simulink model "Kubon_lab6_sim_test"  (R2020a)
settings: Solver=VariableStepAuto  StartTime=0.0  StopTime=10  RelTol=1e-3
values from neighbouring files (symbols this model uses):
  a1 = 1    [Kubon_lab4.m]    (also in Kubon_lab6.m = Aw1*sqrt(2*g/H1); Kubon_lab6_test.m = Aw1*sqrt(2*g/H1); Kubon_lab7.m = Aw1*sqrt(2*g/(H1-H2)); Kubon_lab8.m = Aw1*sqrt(2*g/(H1-H2)))
  A1 = [0,-6/7,-16/7,47/7]    [Kubon_lab4.m]    (also in Kubon_lab6.m = 1; Kubon_lab6_test.m = 1; Kubon_lab7.m = 4; Kubon_lab8.m = 4)
  A2 = 7    [Kubon_lab6.m]    (also in Kubon_lab6_test.m; Kubon_lab7.m = 4; Kubon_lab8.m = 4)
  a2 = Aw2*sqrt(2*g/H2)    [Kubon_lab6.m]    (also in Kubon_lab6_test.m; Kubon_lab7.m; Kubon_lab8.m)
  dfwe1 = 0.1*fwe1max    [Kubon_lab6_test.m]
  dfwe2 = 0.1*fwe2max    [Kubon_lab6_test.m]
  fwe1 = fwe1w(i)    [Kubon_lab6.m]    (also in Kubon_lab6_test.m; Kubon_lab7.m = 0.1*fwe1max; Kubon_lab8.m = 0.1*fwe1max)
  fwe2 = fwe2w(i)    [Kubon_lab6.m]    (also in Kubon_lab6_test.m; Kubon_lab7.m; Kubon_lab8.m)
  h10 = fwe1/a1    [Kubon_lab6.m]    (also in Kubon_lab6_test.m; Kubon_lab7.m = (1/(2*g))*(fwe1/Aw1)^2 + (1/(2*g))*(((fwe2+fwe1)/Aw2)^2); Kubon_lab8.m = fwe1/a1+(fwe2+fwe1)/a2)
  h20 = (fwe1+fwe2)/a2    [Kubon_lab6.m]    (also in Kubon_lab6_test.m; Kubon_lab7.m = 1/(2*g)*(((fwe1+fwe2)/Aw2)^2); Kubon_lab8.m = (fwe2+fwe1)/a2)
  t0 = 50.0    (= 50)    [Kubon_lab10.m]    (also in Kubon_lab4.m = 5; Kubon_lab5.m = 0; Kubon_lab6.m = 5; Kubon_lab6_test.m = 0)
settings Model: Creator=dominika  LastModifiedBy=dominika

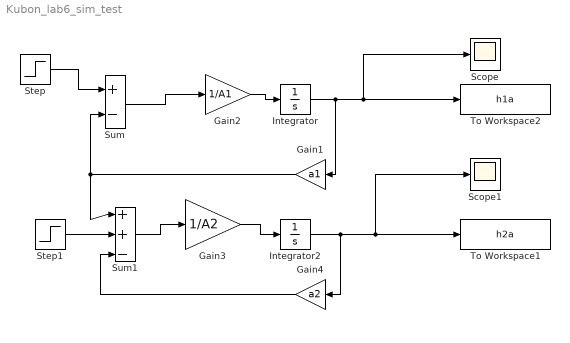
== system Kubon_lab6_sim_test ==
  Gain1 : Gain  Gain=a1
  Gain2 : Gain  Gain=1/A1
  Gain3 : Gain  Gain=1/A2
  Gain4 : Gain  Gain=a2
  Integrator : Integrator  InitialCondition=h10
  Integrator2 : Integrator  InitialCondition=h20
  Scope : Scope
  Scope1 : Scope
  Step : Step  Time=t0  Before=fwe1  After=fwe1+ dfwe1  SampleTime=0
  Step1 : Step  Time=t0  Before=fwe2  After=fwe2+ dfwe2  SampleTime=0
  Sum : Sum  Inputs=+-
  Sum1 : Sum  Inputs=++-
  To Workspace1 : ToWorkspace  VariableName=h2a  SampleTime=-1
  To Workspace2 : ToWorkspace  VariableName=h1a  SampleTime=-1
  wires:
  Sum/1 -> Gain2/1
  Integrator/1 -> Gain1/1, To Workspace2/1, Scope/1
  Gain1/1 -> Sum/2, Sum1/1
  Step/1 -> Sum/1
  Gain2/1 -> Integrator/1
  Sum1/1 -> Gain3/1
  Gain3/1 -> Integrator2/1
  Step1/1 -> Sum1/2
  Integrator2/1 -> Scope1/1, To Workspace1/1, Gain4/1
  Gain4/1 -> Sum1/3
